simulink model "autosar_LaneGuidance"  (R2023b)
settings: Solver=FixedStepAuto  StartTime=0.0  StopTime=10.0  FixedStep=1/10  RelTol=1e-3
model workspace (MAT data in the model file):
  HazardLightsOFF = Simulink.Parameter
  HazardLightsOFF.Value = 0
  HazardLightsOFF.DataType = 'auto'
  HazardLightsOFF.Complexity = 'real'
  HazardLightsOFF.Dimensions = [1 1]
  HazardLightsON = Simulink.Parameter
  HazardLightsON.Value = 1
  HazardLightsON.DataType = 'auto'
  HazardLightsON.Complexity = 'real'
  HazardLightsON.Dimensions = [1 1]
  SafeDistanceThreshold = Simulink.Parameter
  SafeDistanceThreshold.Value = 0.1
  SafeDistanceThreshold.DataType = 'auto'
  SafeDistanceThreshold.Complexity = 'real'
  SafeDistanceThreshold.Dimensions = [1 1]
libraries: autosarlibaprouting x8
settings Model: Creator=The MathWorks, Inc.  LastModifiedBy=The MathWorks, Inc.
settings SolverCC: AlgebraicLoopSolver=TrustRegion
settings DataIOCC: ReturnWorkspaceOutputs=off
settings OptimizationCC: DefaultParameterBehavior=Inlined  EnhancedBackFolding=on  PassReuseOutputArgsAs=Individual arguments  ZeroExternalMemoryAtStartup=off  ZeroInternalMemoryAtStartup=off  OptimizeBlockOrder=speed  DifferentSizesBufferReuse=on  OptimizationCustomize=off  EfficientTunableParamExpr=on
settings DebuggingCC: ParameterTunabilityLossMsg=error  UnconnectedInputMsg=warning  UnconnectedOutputMsg=warning  UnconnectedLineMsg=warning  ArithmeticOperatorsInVariantConditions=warning
settings HardwareCC: ProdBitPerLong=64  ProdHWDeviceType=Intel->x86-64 (Linux 64)
settings ModelReferenceCC: EnableRefExpFcnMdlSchedulingChecks=on
settings SFSimCC: SimUseLocalCustomCode=off  MATLABDynamicMemAlloc=off  CustomCodeUndefinedFunction=UseInterfaceOnly  SimTargetLang=C++
settings RTWCC: Description=AUTOSAR Adaptive  SystemTargetFile=autosar_adaptive.tlc  GenCodeOnly=on  PackageName=mApp.zip  TemplateMakefile=ert_default_tmf  GenerateReport=on  RTWUseLocalCustomCode=off  Toolchain=AUTOSAR Adaptive | CMake  IncludeHyperlinkInReport=on  LaunchReport=on  DataTypeReplacement=CDataTypesFixedWidth  TargetLang=C++  GenerateTraceInfo=on  GenerateTraceReport=on  GenerateTraceReportSl=on  GenerateTraceReportSf=on  GenerateTraceReportEml=on  DLArmComputeVersion=19.05
settings CodeAppCC: ForceParamTrailComments=on  IgnoreCustomStorageClasses=off  MaxIdLength=63  OperatorAnnotations=on  SimulinkDataObjDesc=on  SFDataObjDesc=on  InsertBlockDesc=on
settings AUTOSARAdaptiveTargetCC: TargetFcnLib=ansi_tfl_table_tmw.mat  GenFloatMathFcnCalls=NOT IN USE  TargetLangStandard=C++11 (ISO)  CodeReplacementLibrary=None  UtilityFuncGeneration=Auto  MultiwordTypeDef=System defined  MultiwordLength=2048  DynamicStringBufferSize=256  GenerateFullHeader=on  InferredTypesCompatibility=off  GenerateSampleERTMain=off  GenerateTestInterfaces=off  ModelReferenceCompliant=on  ParMdlRefBuildCompliant=on  CompOptLevelCompliant=on  ConcurrentExecutionCompliant=on  IncludeMdlTerminateFcn=on  CombineOutputUpdateFcns=on  CombineSignalStateStructs=off  GroupInternalDataByFunction=off  SuppressErrorStatus=on  IncludeFileDelimiter=Auto  ERTCustomFileBanners=off  SupportAbsoluteTime=on  LogVarNameModifier=rt_  MatFileLogging=off  CodeInterfacePackaging=C++ class  PurelyIntegerCode=off  SupportNonFinite=off  SupportComplex=on  SupportContinuousTime=off  SupportNonInlinedSFcns=off  RemoveDisableFunc=off  RemoveResetFunc=on  SupportVariableSizeSignals=off  ParenthesesLevel=Nominal  CastingMode=Nominal  MATLABClassNameForMDSCustomization=Simulink.SoftwareTarget.TargetSpecificTriggerConfigurationBase  ModelStepFunctionPrototypeControlCompliant=off  CPPClassGenCompliant=on  AutosarCompliant=on  MDXCompliant=off  GRTInterface=off  GenerateAllocFcn=off  UseToolchainInfoCompliant=on  GenerateSharedConstants=on  CoderGroups=[]  AccessMethods=[]  LookupTableObjectStructAxisOrder=2,1,3,4,...  LUTObjectStructOrderExplicitValues=Size,Breakpoints,Table  LUTObjectStructOrderEvenSpacing=Size,Table,Breakpoints  ArrayLayout=Column-major  UnsupportedSFcnMsg=error  ERTHeaderFileRootName=$R$E  ERTSourceFileRootName=$R$E  ERTDataFileRootName=$R_data  OptimizeReductions=off  GenerateASAP2=off  DSAsUniqueAccess=off  ExtMode=off  ExtModeTransport=0  ExtModeStaticAlloc=off  ExtModeAutomaticAllocSize=on  ExtModeMaxTrigDuration=10  ExtModeStaticAllocSize=1000000  ExtModeTesting=off  ExtModeMexFile=ext_comm  ExtModeIntrfLevel=Level1  InlinedParameterPlacement=NonHierarchical  TargetOS=BareBoardExample  MultiInstanceErrorCode=Error  RootIOFormat=Structure reference  RTWCAPISignals=off  RTWCAPIParams=off  RTWCAPIStates=off  RTWCAPIRootIO=off  ERTSrcFileBannerTemplate=ert_code_template.cgt  ERTHdrFileBannerTemplate=ert_code_template.cgt  ERTDataSrcFileTemplate=ert_code_template.cgt  ERTDataHdrFileTemplate=ert_code_template.cgt  ERTCustomFileTemplate=example_file_process.tlc  EnableDataOwnership=off  SignalDisplayLevel=10  ParamTuneLevel=10  GlobalDataDefinition=Auto  DataDefinitionFile=global.c  GlobalDataReference=Auto  ERTFilePackagingFormat=Compact  RateTransitionBlockCode=Inline  DataReferenceFile=global.h  PreserveExpressionOrder=off  PreserveIfCondition=off  ConvertIfToSwitch=on  PreserveExternInFcnDecls=on  PreserveStaticInFcnDecls=on  SuppressUnreachableDefaultCases=on  EnableSignedLeftShifts=on  EnableSignedRightShifts=on  ImplementImageWithCVMat=off  IndentStyle=K&R  IndentSize=2  NewlineStyle=Default  MaxLineWidth=80  EnableUserReplacementTypes=off  MaxIdInt64=INT64_MAX  MinIdInt64=INT64_MIN  MaxIdUint64=UINT64_MAX  MaxIdInt32=INT32_MAX  MinIdInt32=INT32_MIN  MaxIdUint32=UINT32_MAX  MaxIdInt16=INT16_MAX  MinIdInt16=INT16_MIN  MaxIdUint16=UINT16_MAX  MaxIdInt8=INT8_MAX  MinIdInt8=INT8_MIN  MaxIdUint8=UINT8_MAX  BooleanTrueId=true  BooleanFalseId=false  MemSecPackage=--- None ---  MemSecDataConstants=Default  MemSecDataIO=Default  MemSecDataInternal=Default  MemSecDataParameters=Default  MemSecFuncInitTerm=Default  MemSecFuncExecute=Default  MemSecFuncSharedUtil=Default  GroupConstants=Default  GroupRootInputs=Default  GroupRootOutputs=Default  GroupInternal=Default  GroupParameters=Default  GroupDataTransfer=Default  GroupSharedLocalDataStores=Default  GroupInstanceSpecificParameters=Default  GroupModelData=Default  ArrayContainerType=C-style array  AutosarSchemaVersion=R19-11  AutosarMaxShortNameLength=128  AdaptiveAutosarXCPServerTransportLayer=None  AdaptiveAutosarXCPServerTCPIPAddress=127.0.0.1  AdaptiveAutosarXCPServerPort=17725  AdaptiveAutosarXCPServerVerbosity=off  AdaptiveAutosarUseCustomXCPServer=off

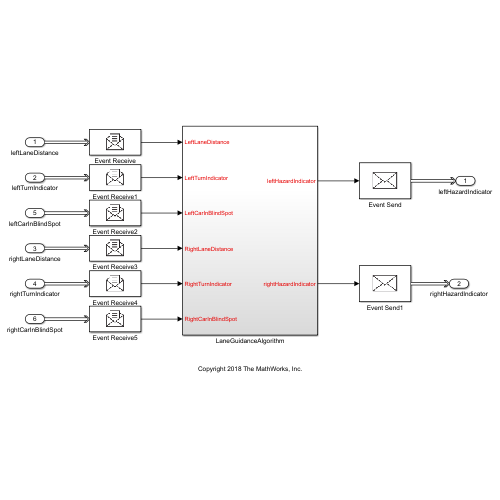
[thumbnail: Simulink's stored preview of the top-level diagram]
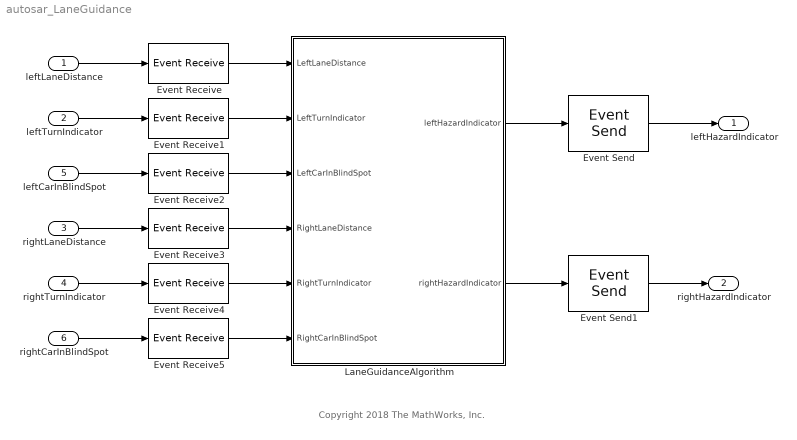
== system autosar_LaneGuidance ==
  note: Copyright 2018 The MathWorks, Inc.
  leftLaneDistance : Inport  OutputPortMessageModes=m  OutDataTypeStr=double  PortDimensions=1
  leftTurnIndicator : Inport  OutputPortMessageModes=m  Port=2  OutDataTypeStr=double  PortDimensions=1
  rightLaneDistance : Inport  OutputPortMessageModes=m  Port=3  OutDataTypeStr=double  PortDimensions=1
  rightTurnIndicator : Inport  OutputPortMessageModes=m  Port=4  OutDataTypeStr=double  PortDimensions=1
  leftCarInBlindSpot : Inport  OutputPortMessageModes=m  Port=5  OutDataTypeStr=double  PortDimensions=1
  rightCarInBlindSpot : Inport  OutputPortMessageModes=m  Port=6  OutDataTypeStr=double  PortDimensions=1
  Event Receive{,1..5} (6 alike) : autosarlibaprouting/Event Receive
  Event Send : autosarlibaprouting/Event Send
  Event Send1 : autosarlibaprouting/Event Send
  LaneGuidanceAlgorithm : Subsystem
  leftHazardIndicator : Outport  InputPortMessageModes=m  OutDataTypeStr=double  PortDimensions=1  VectorParamsAs1DForOutWhenUnconnected=off
  rightHazardIndicator : Outport  InputPortMessageModes=m  Port=2  OutDataTypeStr=double  PortDimensions=1  VectorParamsAs1DForOutWhenUnconnected=off
  wires:
  leftLaneDistance/1 -> Event Receive/1
  Event Receive/1 -> LaneGuidanceAlgorithm/1(LeftLaneDistance)
  leftTurnIndicator/1 -> Event Receive1/1
  Event Receive1/1 -> LaneGuidanceAlgorithm/2(LeftTurnIndicator)
  leftCarInBlindSpot/1 -> Event Receive2/1
  Event Receive2/1 -> LaneGuidanceAlgorithm/3(LeftCarInBlindSpot)
  rightLaneDistance/1 -> Event Receive3/1
  Event Receive3/1 -> LaneGuidanceAlgorithm/4(RightLaneDistance)
  rightTurnIndicator/1 -> Event Receive4/1
  rightCarInBlindSpot/1 -> Event Receive5/1
  Event Receive4/1 -> LaneGuidanceAlgorithm/5(RightTurnIndicator)
  Event Receive5/1 -> LaneGuidanceAlgorithm/6(RightCarInBlindSpot)
  LaneGuidanceAlgorithm/1(leftHazardIndicator) -> Event Send/1
  Event Send/1 -> leftHazardIndicator/1
  LaneGuidanceAlgorithm/2(rightHazardIndicator) -> Event Send1/1
  Event Send1/1 -> rightHazardIndicator/1

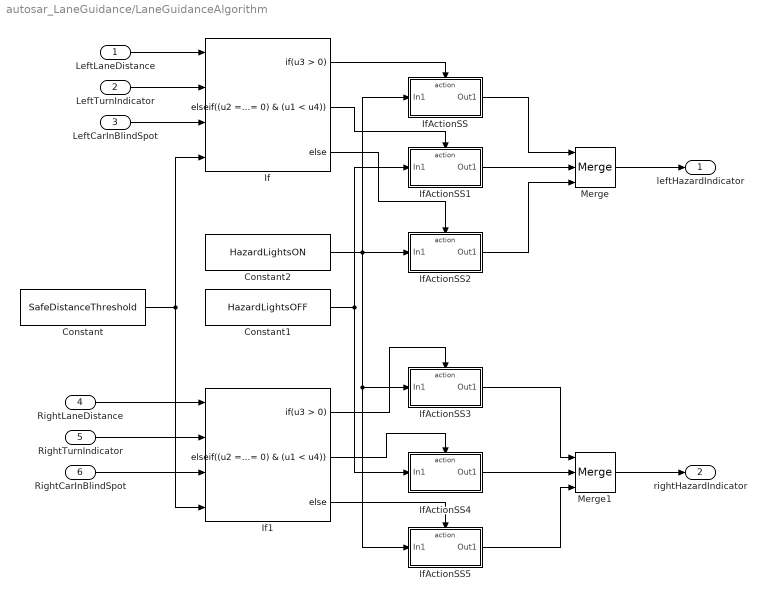
== system autosar_LaneGuidance/LaneGuidanceAlgorithm ==
  LeftLaneDistance : Inport
  LeftTurnIndicator : Inport  Port=2
  LeftCarInBlindSpot : Inport  Port=3
  RightLaneDistance : Inport  Port=4
  RightTurnIndicator : Inport  Port=5
  RightCarInBlindSpot : Inport  Port=6
  Constant : Constant  Value=SafeDistanceThreshold
  Constant1 : Constant  Value=HazardLightsOFF
  Constant2 : Constant  Value=HazardLightsON
  If : If  NumInputs=4  IfExpression=u3 > 0  ElseIfExpressions=(u2 == 0) & (u1 < u4)
  If1 : If  NumInputs=4  IfExpression=u3 > 0  ElseIfExpressions=(u2 == 0) & (u1 < u4)
  IfActionSS : Subsystem  TreatAsAtomicUnit=on
  IfActionSS1 : Subsystem  TreatAsAtomicUnit=on
  IfActionSS2 : Subsystem  TreatAsAtomicUnit=on
  IfActionSS3 : Subsystem  TreatAsAtomicUnit=on
  IfActionSS4 : Subsystem  TreatAsAtomicUnit=on
  IfActionSS5 : Subsystem  TreatAsAtomicUnit=on
  Merge : Merge  Inputs=3
  Merge1 : Merge  Inputs=3
  leftHazardIndicator : Outport  VectorParamsAs1DForOutWhenUnconnected=off
  rightHazardIndicator : Outport  Port=2  VectorParamsAs1DForOutWhenUnconnected=off
  wires:
  Merge/1 -> leftHazardIndicator/1
  If/3 -> IfActionSS2/Action
  Constant/1 -> If/4, If1/4
  LeftCarInBlindSpot/1 -> If/3
  LeftTurnIndicator/1 -> If/2
  LeftLaneDistance/1 -> If/1
  IfActionSS2/1(Out1) -> Merge/3
  IfActionSS1/1(Out1) -> Merge/2
  IfActionSS/1(Out1) -> Merge/1
  If/1 -> IfActionSS/Action
  If/2 -> IfActionSS1/Action
  Constant2/1 -> IfActionSS5/1(In1), IfActionSS3/1(In1), IfActionSS/1(In1), IfActionSS2/1(In1)
  Constant1/1 -> IfActionSS4/1(In1), IfActionSS1/1(In1)
  If1/2 -> IfActionSS4/Action
  If1/1 -> IfActionSS3/Action
  IfActionSS3/1(Out1) -> Merge1/1
  IfActionSS4/1(Out1) -> Merge1/2
  IfActionSS5/1(Out1) -> Merge1/3
  If1/3 -> IfActionSS5/Action
  Merge1/1 -> rightHazardIndicator/1
  RightLaneDistance/1 -> If1/1
  RightTurnIndicator/1 -> If1/2
  RightCarInBlindSpot/1 -> If1/3

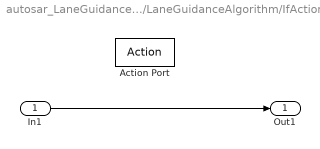
== system autosar_LaneGuidance/LaneGuidanceAlgorithm/IfActionSS ==
  In1 : Inport
  Action Port : ActionPort  ActionPortLabel=if(u3 > 0)
  Out1 : Outport  VectorParamsAs1DForOutWhenUnconnected=off
  wires:
  In1/1 -> Out1/1

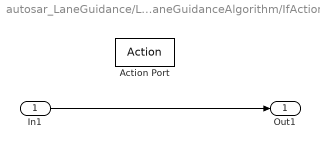
== system autosar_LaneGuidance/LaneGuidanceAlgorithm/IfActionSS1 ==
  In1 : Inport
  Action Port : ActionPort  ActionPortLabel=elseif((u2 == 0) & (u1 < u4))
  Out1 : Outport  VectorParamsAs1DForOutWhenUnconnected=off
  wires:
  In1/1 -> Out1/1

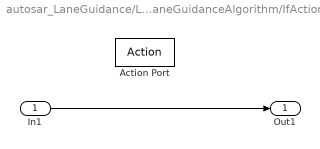
== system autosar_LaneGuidance/LaneGuidanceAlgorithm/IfActionSS2 ==
  In1 : Inport
  Action Port : ActionPort  ActionPortLabel=else
  Out1 : Outport  VectorParamsAs1DForOutWhenUnconnected=off
  wires:
  In1/1 -> Out1/1

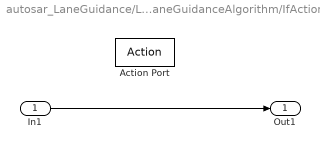
== system autosar_LaneGuidance/LaneGuidanceAlgorithm/IfActionSS3 ==
  In1 : Inport
  Action Port : ActionPort  ActionPortLabel=if(u3 > 0)
  Out1 : Outport  VectorParamsAs1DForOutWhenUnconnected=off
  wires:
  In1/1 -> Out1/1

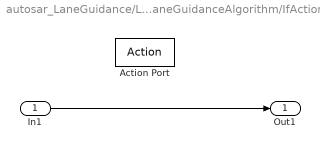
== system autosar_LaneGuidance/LaneGuidanceAlgorithm/IfActionSS4 ==
  In1 : Inport
  Action Port : ActionPort  ActionPortLabel=elseif((u2 == 0) & (u1 < u4))
  Out1 : Outport  VectorParamsAs1DForOutWhenUnconnected=off
  wires:
  In1/1 -> Out1/1

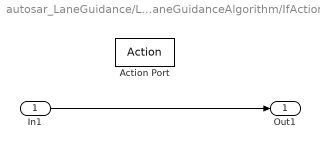
== system autosar_LaneGuidance/LaneGuidanceAlgorithm/IfActionSS5 ==
  In1 : Inport
  Action Port : ActionPort  ActionPortLabel=else
  Out1 : Outport  VectorParamsAs1DForOutWhenUnconnected=off
  wires:
  In1/1 -> Out1/1
